simulink model "achando_relacao_hall_convencao_zero"  (R2012b)
settings: Solver=ode45  StartTime=0.0  StopTime=1  RelTol=1e-3
libraries: BLDC x3, simulink x1
settings Model: Creator=Juliano  LastModifiedBy=Juliano

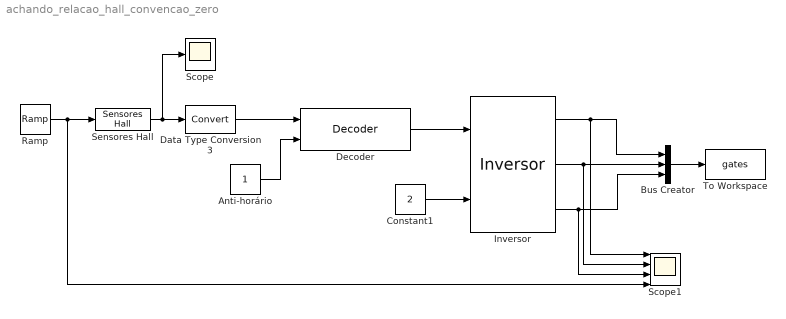
== system achando_relacao_hall_convencao_zero ==
  Anti-horário : Constant
  Bus Creator : BusCreator  Inputs=3
  Constant1 : Constant  Value=2
  Data Type Conversion3 : DataTypeConversion  SaturateOnIntegerOverflow=on  RndMeth=Zero
  Decoder : BLDC/BLDC (block commutation)/Decoder
  Inversor : BLDC/BLDC (block commutation)/Inversor
  Ramp : simulink/Sources/Ramp  slope=2*pi  start=0  X0=0
  Scope : Scope
  Scope1 : Scope  NumInputPorts=4
      settings: YMin=-2~-2~-2~-5  YMax=2~2~2~5
  Sensores Hall : BLDC/BLDC (block commutation)/Sensores Hall
  To Workspace : ToWorkspace  VariableName=gates  SampleTime=-1
  wires:
  Sensores Hall/1 -> Scope/1, Data Type Conversion3/1
  Data Type Conversion3/1 -> Decoder/1
  Anti-horário/1 -> Decoder/2
  Decoder/1 -> Inversor/1
  Ramp/1 -> Scope1/4, Sensores Hall/1
  Constant1/1 -> Inversor/2
  Inversor/1 -> Scope1/1, Bus Creator/1
  Inversor/2 -> Scope1/2, Bus Creator/2
  Inversor/3 -> Bus Creator/3, Scope1/3
  Bus Creator/1 -> To Workspace/1
